simulink model "counter_w_enable_reset"  (R2012b)
settings: Solver=ode45  StartTime=0.0  StopTime=10.0  RelTol=1e-3
libraries: simulink x1
settings Model: Creator=Carl  LastModifiedBy=Carl

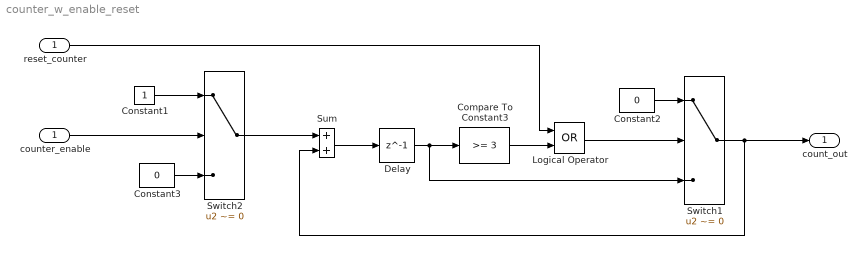
== system counter_w_enable_reset ==
  reset_counter : Inport
  Compare To Constant3 : simulink/Logic and Bit Operations/Compare To Constant  relop=>=  const=3  OutDataTypeStr=boolean  ZeroCross=off
  Constant1 : Constant  OutDataTypeStr=uint32
  Constant2 : Constant  Value=0  OutDataTypeStr=uint32
  Constant3 : Constant  Value=0  OutDataTypeStr=uint32
  Delay : Delay  DelayLength=1  InitialCondition=0
  Logical Operator : Logic  Operator=OR  AllPortsSameDT=off  OutDataTypeStr=boolean
  Sum : Sum  OutDataTypeStr=uint32  RndMeth=Nearest  SaturateOnIntegerOverflow=on
  Switch1 : Switch  Criteria=u2 ~= 0
  Switch2 : Switch  Criteria=u2 ~= 0
  counter_enable : InportShadow
  count_out : Outport
  wires:
  Switch1/1 -> Sum/2, count_out/1
  Delay/1 -> Compare To Constant3/1, Switch1/3
  Constant2/1 -> Switch1/1
  Logical Operator/1 -> Switch1/2
  Compare To Constant3/1 -> Logical Operator/2
  reset_counter/1 -> Logical Operator/1
  Sum/1 -> Delay/1
  Switch2/1 -> Sum/1
  counter_enable/1 -> Switch2/2
  Constant1/1 -> Switch2/1
  Constant3/1 -> Switch2/3
